simulink model "Quarter_car_suspension"  (R2020a)
settings: Solver=VariableStepAuto  StartTime=0.0  StopTime=10.0  RelTol=1e-3
undefined symbols (not defined in the file): c_com, c_re, k1, k2, mc, ms, v
settings Model: Creator=naina  LastModifiedBy=naina

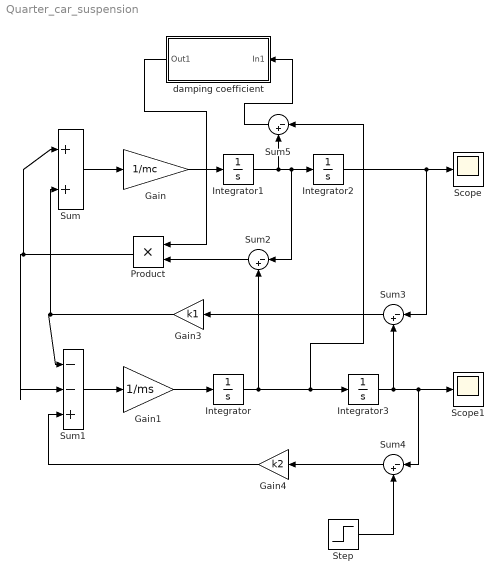
== system Quarter_car_suspension ==
  Gain : Gain  Gain=1/mc
  Gain1 : Gain  Gain=1/ms
  Gain3 : Gain  Gain=k1
  Gain4 : Gain  Gain=k2
  Integrator{,1..3} (4 alike) : Integrator
  Product : Product
  Scope : Scope
  Scope1 : Scope
  Step : Step  After=30  SampleTime=0
  Sum : Sum  Inputs=|++
  Sum1 : Sum  Inputs=|--+
  Sum{2..5} (4 alike) : Sum  Inputs=|-+
  damping coefficient : Subsystem
  wires:
  Sum/1 -> Gain/1
  Gain/1 -> Integrator1/1
  Integrator1/1 -> Sum5/2, Sum2/1, Integrator2/1
  Sum1/1 -> Gain1/1
  Gain1/1 -> Integrator/1
  Integrator/1 -> Sum5/1, Integrator3/1, Sum2/2
  Integrator3/1 -> Scope1/1, Sum4/1, Sum3/2
  Step/1 -> Sum4/2
  Sum4/1 -> Gain4/1
  Gain4/1 -> Sum1/3
  Sum3/1 -> Gain3/1
  Sum2/1 -> Product/2
  Integrator2/1 -> Sum3/1, Scope/1
  Sum5/1 -> damping coefficient/1(In1)
  damping coefficient/1(Out1) -> Product/1
  Gain3/1 -> Sum/2, Sum1/1
  Product/1 -> Sum/1, Sum1/2

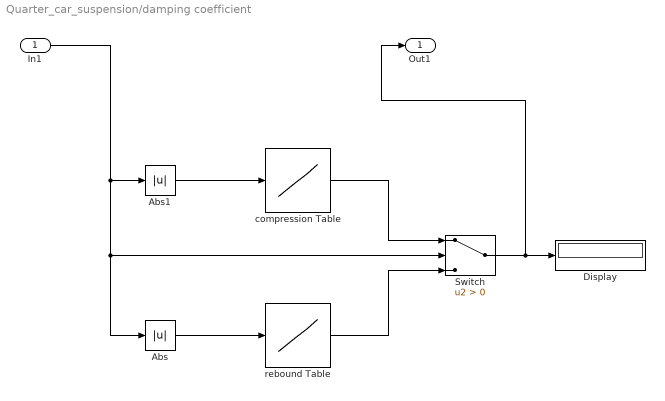
== system Quarter_car_suspension/damping coefficient ==
  In1 : Inport
  Abs : Abs
  Abs1 : Abs
  Display : Display
  Switch : Switch  Criteria=u2 > Threshold
  compression Table : Lookup_n-D  NumberOfTableDimensions=1  BreakpointsForDimension1=v  Table=c_com  InternalRulePriority=Speed  RndMeth=Simplest  InputSameDT=on
  rebound Table : Lookup_n-D  NumberOfTableDimensions=1  BreakpointsForDimension1=v  Table=c_re  InternalRulePriority=Speed  RndMeth=Simplest  InputSameDT=on
  Out1 : Outport
  wires:
  Abs/1 -> rebound Table/1
  Abs1/1 -> compression Table/1
  In1/1 -> Abs/1, Switch/2, Abs1/1
  compression Table/1 -> Switch/1
  rebound Table/1 -> Switch/3
  Switch/1 -> Out1/1, Display/1
